simulink model "six"  (R2020b)
settings: Solver=VariableStepAuto  StartTime=0.0  StopTime=10.0  RelTol=1e-3
settings Model: Creator=USER  LastModifiedBy=USER

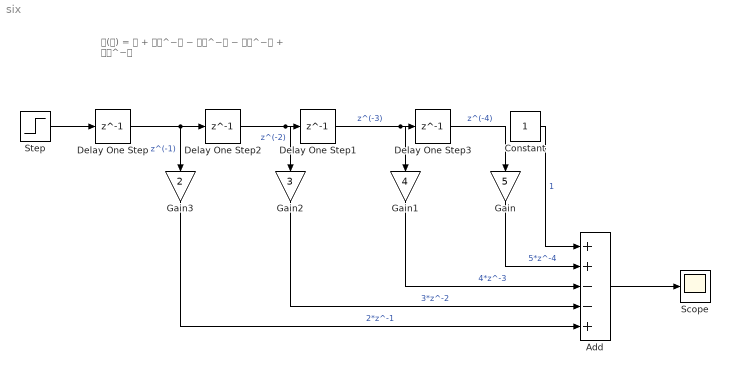
== system six ==
  note: 𝐇(𝐳) = 𝟏 + 𝟐𝐳^−𝟏 − 𝟑𝐳^−𝟐 − 𝟒𝐳^−𝟑 + 𝟓𝐳^−𝟒
  Add : Sum  Inputs=++--+
  Constant : Constant
  Delay One Step{,1..3} (4 alike) : Delay  DelayLength=1
  Gain : Gain  Gain=5
  Gain1 : Gain  Gain=4
  Gain2 : Gain  Gain=3
  Gain3 : Gain  Gain=2
  Scope : Scope
  Step : Step  SampleTime=0
  wires:
  Step/1 -> Delay One Step/1
  Delay One Step2/1 -> Gain2/1, Delay One Step1/1  "z^(-2)"
  Delay One Step/1 -> Gain3/1, Delay One Step2/1  "z^(-1)"
  Delay One Step1/1 -> Gain1/1, Delay One Step3/1  "z^(-3)"
  Delay One Step3/1 -> Gain/1  "z^(-4)"
  Gain/1 -> Add/2  "5*z^-4"
  Gain1/1 -> Add/3  "4*z^-3"
  Gain2/1 -> Add/4  "3*z^-2"
  Gain3/1 -> Add/5  "2*z^-1"
  Add/1 -> Scope/1
  Constant/1 -> Add/1  "1"
